simulink model "zh1"  (R2024b)
settings: Solver=VariableStepAuto  StartTime=0.0  StopTime=20  RelTol=1e-3
libraries: cstblocks x4

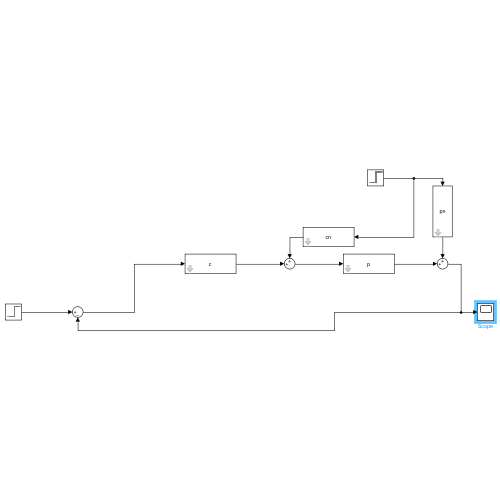
[thumbnail: Simulink's stored preview of the top-level diagram]
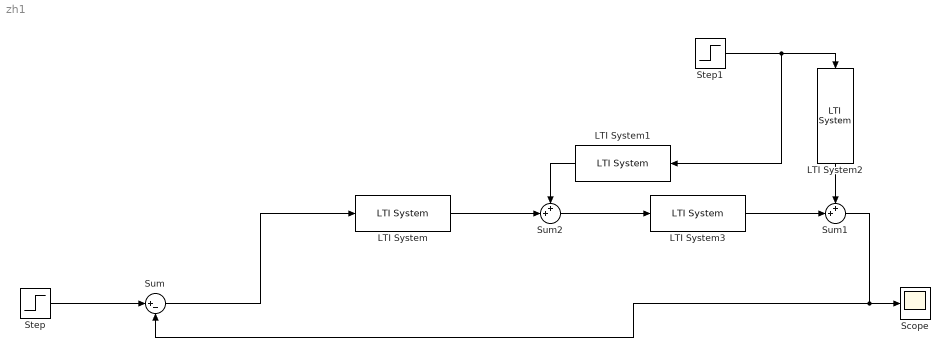
== system zh1 ==
  LTI System : cstblocks/LTI System  sys=c  IC=[]  PadeOrder=0
  LTI System1 : cstblocks/LTI System  sys=cn  IC=[]  PadeOrder=0
  LTI System2 : cstblocks/LTI System  sys=pn  IC=[]  PadeOrder=0
  LTI System3 : cstblocks/LTI System  sys=p  IC=[]  PadeOrder=0
  Scope : Scope
  Step : Step  SampleTime=0
  Step1 : Step  Time=5  SampleTime=10
  Sum : Sum  Inputs=|+-
  Sum1 : Sum  Inputs=++|
  Sum2 : Sum  Inputs=++|
  wires:
  Sum/1 -> LTI System/1
  Step/1 -> Sum/1
  Sum1/1 -> Sum/2, Scope/1
  LTI System/1 -> Sum2/2
  LTI System1/1 -> Sum2/1
  Step1/1 -> LTI System1/1, LTI System2/1
  LTI System2/1 -> Sum1/1
  Sum2/1 -> LTI System3/1
  LTI System3/1 -> Sum1/2
